simulink model "tarea1"  (R2026a)
settings: Solver=ode45  StartTime=0.001
settings Model: Creator=jmlc2  LastModifiedBy=jmlc2

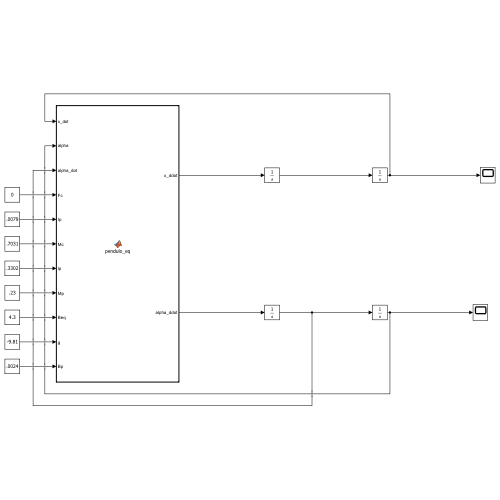
[thumbnail: Simulink's stored preview of the top-level diagram]
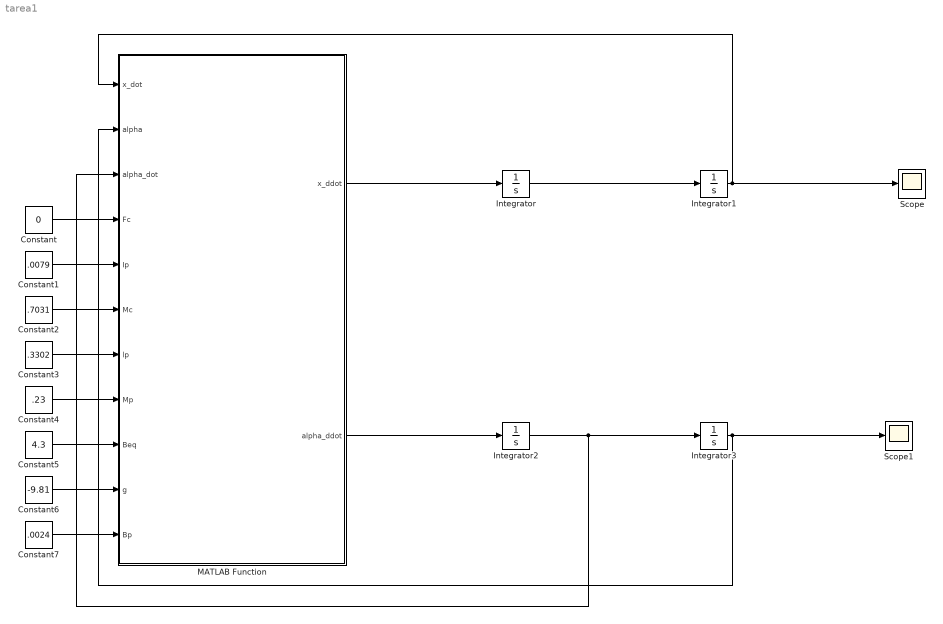
== system tarea1 ==
  Constant : Constant  Value=0
  Constant1 : Constant  Value=.0079
  Constant2 : Constant  Value=.7031
  Constant3 : Constant  Value=.3302
  Constant4 : Constant  Value=.23
  Constant5 : Constant  Value=4.3
  Constant6 : Constant  Value=-9.81
  Constant7 : Constant  Value=.0024
  Integrator : Integrator
  Integrator1 : Integrator
  Integrator2 : Integrator
  Integrator3 : Integrator  InitialCondition=pi/180
  MATLAB Function : MATLAB Function  TreatAsAtomicUnit=on
  Scope : Scope
      settings: ActiveDisplayYMinimum=-0.0035062850747050842  ActiveDisplayYMaximum=0.0036535628348446547
  Scope1 : Scope
      settings: ActiveDisplayYMinimum=-0.021289601295778636  ActiveDisplayYMaximum=0.022737616889824112
  wires:
  Constant/1 -> MATLAB Function/4(Fc)
  Constant1/1 -> MATLAB Function/5(Ip)
  Constant2/1 -> MATLAB Function/6(Mc)
  Constant3/1 -> MATLAB Function/7(lp)
  Constant4/1 -> MATLAB Function/8(Mp)
  Constant5/1 -> MATLAB Function/9(Beq)
  Constant6/1 -> MATLAB Function/10(g)
  Constant7/1 -> MATLAB Function/11(Bp)
  MATLAB Function/1(x_ddot) -> Integrator/1
  Integrator/1 -> Integrator1/1
  Integrator1/1 -> MATLAB Function/1(x_dot), Scope/1
  MATLAB Function/2(alpha_ddot) -> Integrator2/1
  Integrator2/1 -> Integrator3/1, MATLAB Function/3(alpha_dot)
  Integrator3/1 -> MATLAB Function/2(alpha), Scope1/1

== matlab function tarea1/MATLAB Function ==
  data: x_dot input; x_ddot output; alpha input; alpha_dot input; Fc input; Ip input; Mc input; lp input; Mp input; Beq input; g input; Bp input; alpha_ddot output
function [x_ddot, alpha_ddot] = pendulo_eq(x_dot, alpha, alpha_dot, Fc, Ip, Mc, lp, Mp, Beq, g, Bp)
M = Mc + Mp;
I_tot = Ip + Mp*lp^2;
den = M * I_tot - (Mp * lp * cos(alpha))^2;
f1 = Fc - Beq*x_dot + Mp*lp*(alpha_dot^2)*sin(alpha);
f2 = Mp*g*lp*sin(alpha) - Bp*alpha_dot;
x_ddot = (I_tot * f1 - Mp*lp*cos(alpha) * f2) / den;
alpha_ddot = (M * f2 - Mp*lp*cos(alpha) * f1) / den;

end
